simulink model "lqrGantryCrane"  (R2017a)
settings: Solver=VariableStepAuto  StartTime=0.0  StopTime=10.0  FixedStep=0.1  RelTol=1e-3
values from neighbouring files (symbols this model uses):
  A =     [GantryModel.mat]
  B = [0 0.5 0 -1]    [GantryModel.mat]
undefined symbols (not defined in the file or in its folder): C, K_lqr, N_lqr
settings Model: Creator=Daniel  LastModifiedBy=Daniel

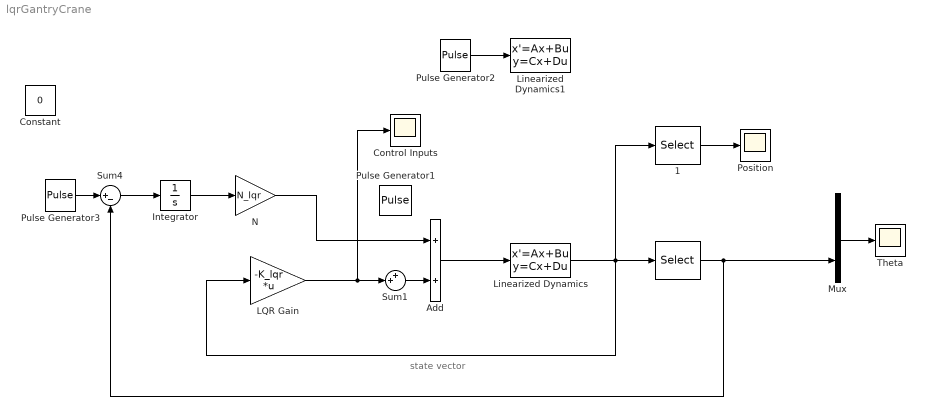
== system lqrGantryCrane ==
  note: state vector
  " " : Selector  InputPortWidth=4  IndexOptions=Index vector (dialog)  Indices=3  OutputSizes=1
  " 1" : Selector  InputPortWidth=4  IndexOptions=Index vector (dialog)  Indices=1  OutputSizes=1
  Add : Sum
  Constant : Constant  Value=0
  Control Inputs : Scope
  Integrator : Integrator
  LQR Gain : Gain  Gain=-K_lqr  Multiplication=Matrix(K*u)  SaturateOnIntegerOverflow=on  OutDataTypeStr=Inherit: Same as input  ParamDataTypeStr=Inherit: Same as input
  Linearized Dynamics : StateSpace  A=A  B=B  C=eye(4)  D=zeros(4,1)  X0=0
  Linearized Dynamics1 : StateSpace  A=A  B=B  C=C  D=0  X0=0
  Mux : Mux  Inputs=2
  N : Gain  Gain=N_lqr
  Position : Scope
  Pulse Generator1 : DiscretePulseGenerator  PulseType=Time based  Period=20  PulseWidth=5
  Pulse Generator2 : DiscretePulseGenerator  PulseType=Time based  Period=20  PulseWidth=5
  Pulse Generator3 : DiscretePulseGenerator  PulseType=Time based  Period=20  PulseWidth=50
  Sum1 : Sum  Inputs=++|
  Sum4 : Sum  Inputs=|+-  SaturateOnIntegerOverflow=on  InputSameDT=on  OutDataTypeStr=Inherit: Same as first input
  Theta : Scope
  wires:
  N/1 -> Add/1
  LQR Gain/1 -> Sum1/2, Control Inputs/1
  Linearized Dynamics/1 -> LQR Gain/1, " "/1, " 1"/1
  Add/1 -> Linearized Dynamics/1
  " 1"/1 -> Position/1
  Sum1/1 -> Add/2
  Pulse Generator2/1 -> Linearized Dynamics1/1
  " "/1 -> Sum4/2, Mux/2
  Mux/1 -> Theta/1
  Pulse Generator3/1 -> Sum4/1
  Sum4/1 -> Integrator/1
  Integrator/1 -> N/1
